simulink model "problem4"  (R2023a)
settings: Solver=VariableStepAuto  StartTime=0.0  StopTime=10.0  RelTol=1e-3
libraries: simulink x3
settings Model: Creator=jackr  LastModifiedBy=jackr

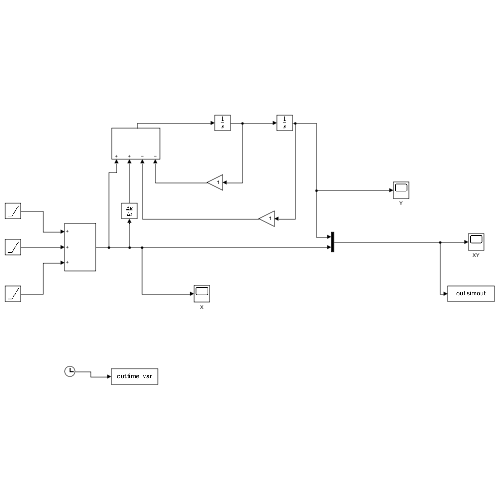
[thumbnail: Simulink's stored preview of the top-level diagram]
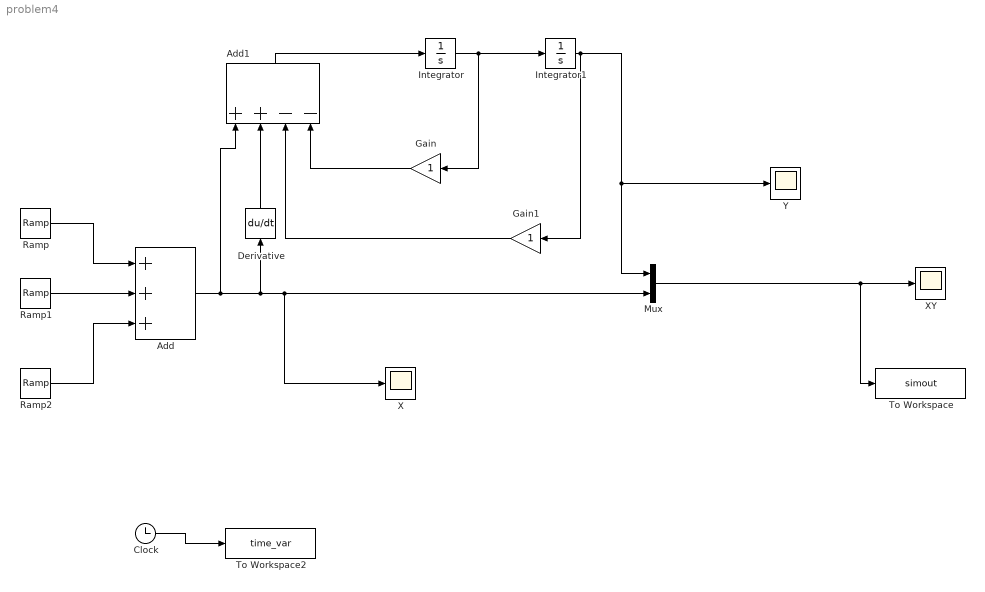
== system problem4 ==
  Add : Sum  Inputs=+++
  Add1 : Sum  Inputs=++--
  Clock : Clock
  Derivative : Derivative
  Gain : Gain
  Gain1 : Gain
  Integrator : Integrator
  Integrator1 : Integrator
  Mux : Mux  Inputs=2
  Ramp : simulink/Sources/Ramp  slope=1  start=0  InitialOutput=0
  Ramp1 : simulink/Sources/Ramp  slope=-2  start=1  InitialOutput=2
  Ramp2 : simulink/Sources/Ramp  slope=1  start=2  InitialOutput=-2
  To Workspace : ToWorkspace  VariableName=simout  SaveFormat=Timeseries  SampleTime=-1
  To Workspace2 : ToWorkspace  VariableName=time_var  SaveFormat=Timeseries  SampleTime=-1
  X : Scope
  XY : Scope
  Y : Scope
  wires:
  Mux/1 -> To Workspace/1, XY/1
  Ramp1/1 -> Add/2
  Integrator/1 -> Gain/1, Integrator1/1
  Integrator1/1 -> Gain1/1, Mux/1, Y/1
  Ramp2/1 -> Add/3
  Ramp/1 -> Add/1
  Add1/1 -> Integrator/1
  Add/1 -> Add1/1, Derivative/1, X/1, Mux/2
  Gain/1 -> Add1/4
  Gain1/1 -> Add1/3
  Derivative/1 -> Add1/2
  Clock/1 -> To Workspace2/1
